simulink model "prob49_e_integral"  (R2016b)
settings: Solver=ode4  StartTime=0.0  StopTime=500.0  FixedStep=0.001  RelTol=1e-3
values from neighbouring files (symbols this model uses):
  alfa = 1    [p49Consts.m]
  beta = 0.1    [p49Consts.m]    (also in task49.m)
  beta_g = 0.1    [p49Consts.m]
  Gamma = [10 0 0 ... (first row only)    [p49Consts.m]
  k = 5    [p49Consts.m]    (also in task49.m)
  lambda_0 = 4    [p49Consts.m]    (also in task49.m = 1)
  lambda_1 = 4    [p49Consts.m]    (also in task49.m = 1)
settings Model: Creator=Kristian  LastModifiedBy=Kristian

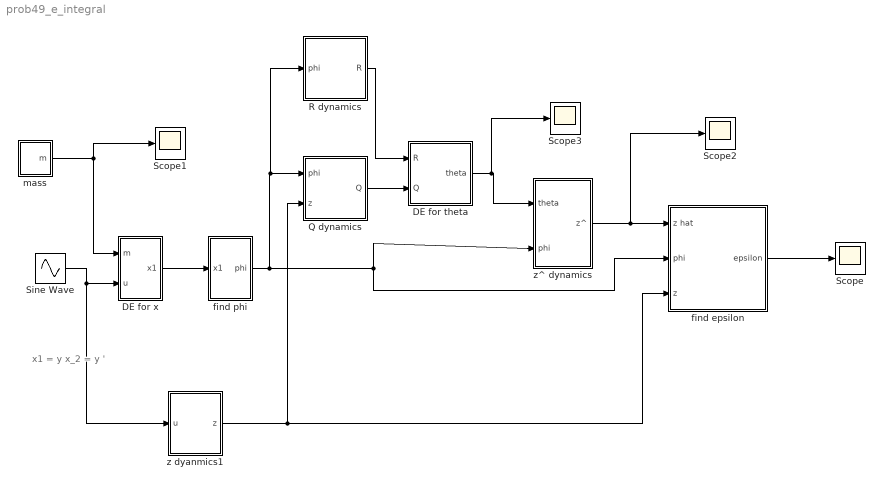
== system prob49_e_integral ==
  note: x1 = y
      | x_2 = y '
  DE for theta : Subsystem
  DE for x : Subsystem
  "Q dynamics " : Subsystem
  "R dynamics " : Subsystem
  Scope{,1..3} (4 alike) : Scope
  Sine Wave : Sin  Amplitude=5  Phase=0.3  SampleTime=0
  find epsilon : Subsystem
  find phi : Subsystem
  "mass " : Subsystem
  z dyanmics1 : Subsystem
  z^ dynamics : Subsystem
  wires:
  DE for x/1("x1 ") -> find phi/1(x1)
  find phi/1("phi ") -> "R dynamics "/1(phi), "Q dynamics "/1(phi), find epsilon/2(phi), z^ dynamics/2(phi)
  Sine Wave/1 -> z dyanmics1/1(u), DE for x/2(u)
  z^ dynamics/1("z^ ") -> Scope2/1, find epsilon/1(z hat)
  DE for theta/1("theta ") -> Scope3/1, z^ dynamics/1(theta)
  find epsilon/1("epsilon ") -> Scope/1
  z dyanmics1/1("z ") -> find epsilon/3(z), "Q dynamics "/2("z ")
  "Q dynamics "/1(Q) -> DE for theta/2(Q)
  "R dynamics "/1("R ") -> DE for theta/1("R ")
  "mass "/1(m) -> Scope1/1, DE for x/1("m ")

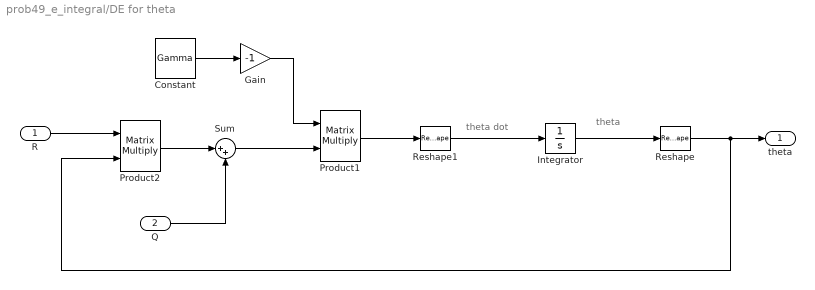
== system prob49_e_integral/DE for theta ==
  note: theta
  note: theta dot
  "R " : Inport
  Q : Inport  Port=2
  Constant : Constant  Value=Gamma  VectorParams1D=off
  Gain : Gain  Gain=-1
  Integrator : Integrator
  Product1 : Product  Multiplication=Matrix(*)
  Product2 : Product  Multiplication=Matrix(*)
  Reshape : Reshape  OutputDimensionality=Column vector (2-D)
  Reshape1 : Reshape  OutputDimensionality=Column vector (2-D)
  Sum : Sum  Inputs=|++
  "theta " : Outport
  wires:
  Integrator/1 -> Reshape/1
  Constant/1 -> Gain/1
  Product1/1 -> Reshape1/1
  Reshape1/1 -> Integrator/1
  Gain/1 -> Product1/1
  "R "/1 -> Product2/1
  Reshape/1 -> Product2/2, "theta "/1
  Product2/1 -> Sum/1
  Q/1 -> Sum/2
  Sum/1 -> Product1/2

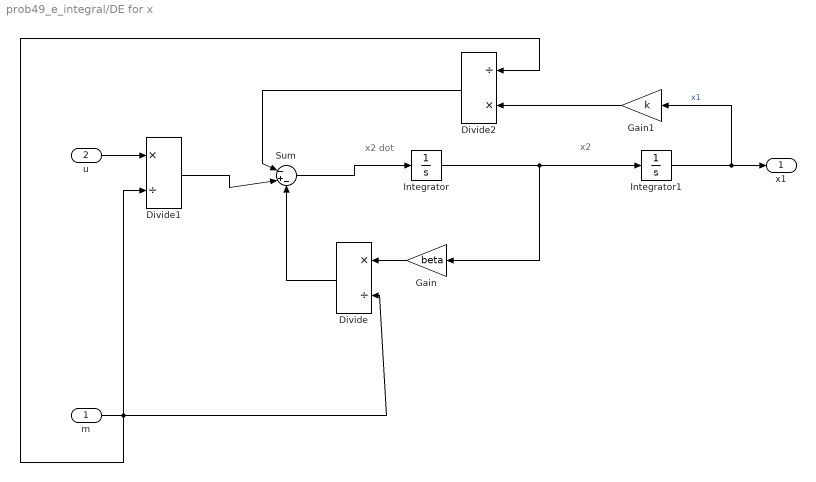
== system prob49_e_integral/DE for x ==
  note: x2 dot
  note: x2
  "m " : Inport
  u : Inport  Port=2
  Divide : Product  Inputs=*/
  Divide1 : Product  Inputs=*/
  Divide2 : Product  Inputs=/*
  Gain : Gain  Gain=beta
  Gain1 : Gain  Gain=k
  Integrator : Integrator
  Integrator1 : Integrator
  Sum : Sum  Inputs=|-+-
  "x1 " : Outport
  wires:
  Integrator/1 -> Integrator1/1, Gain/1
  Sum/1 -> Integrator/1
  Integrator1/1 -> Gain1/1, "x1 "/1  "x1"
  Gain/1 -> Divide/1
  "m "/1 -> Divide2/1, Divide/2, Divide1/2
  u/1 -> Divide1/1
  Gain1/1 -> Divide2/2
  Divide2/1 -> Sum/1
  Divide1/1 -> Sum/2
  Divide/1 -> Sum/3

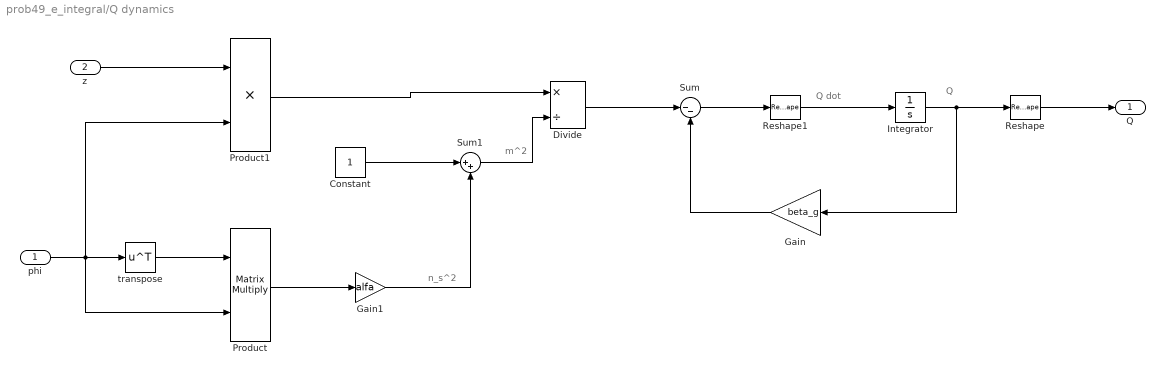
== system prob49_e_integral/Q dynamics  ==
  note: Q
  note: Q dot
  note: n_s^2
  note: m^2
  phi : Inport
  "z " : Inport  Port=2
  Constant : Constant
  Divide : Product  Inputs=*/
  Gain : Gain  Gain=beta_g
  Gain1 : Gain  Gain=alfa
  Integrator : Integrator
  Product : Product  Multiplication=Matrix(*)
  Product1 : Product
  Reshape : Reshape  OutputDimensionality=Column vector (2-D)
  Reshape1 : Reshape  OutputDimensionality=Column vector (2-D)
  Sum : Sum  Inputs=|--
  Sum1 : Sum  Inputs=|++
  transpose : Math  Operator=transpose  SaturateOnIntegerOverflow=on
  Q : Outport
  wires:
  Integrator/1 -> Gain/1, Reshape/1
  Reshape1/1 -> Integrator/1
  Reshape/1 -> Q/1
  Gain/1 -> Sum/2
  Sum/1 -> Reshape1/1
  Constant/1 -> Sum1/1
  transpose/1 -> Product/1
  Product/1 -> Gain1/1
  Gain1/1 -> Sum1/2
  phi/1 -> Product1/2, Product/2, transpose/1
  Product1/1 -> Divide/1
  Sum1/1 -> Divide/2
  Divide/1 -> Sum/1
  "z "/1 -> Product1/1

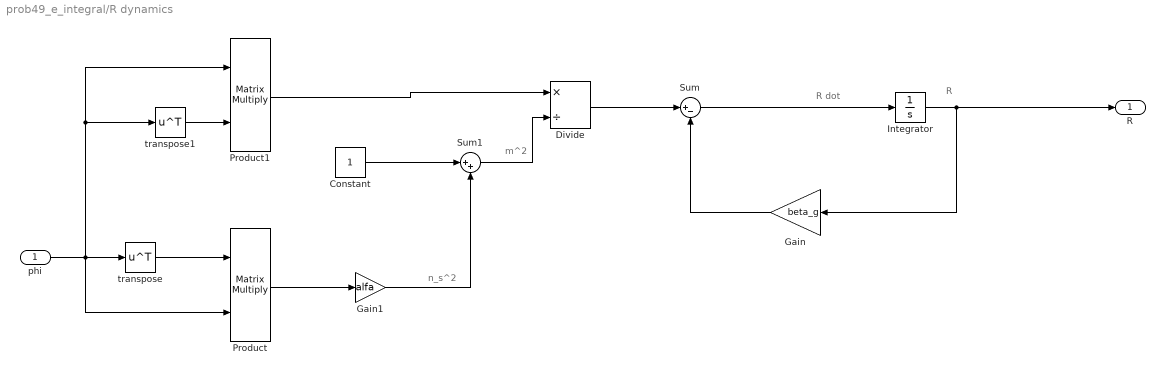
== system prob49_e_integral/R dynamics  ==
  note: R
  note: R dot
  note: n_s^2
  note: m^2
  phi : Inport
  Constant : Constant
  Divide : Product  Inputs=*/
  Gain : Gain  Gain=beta_g
  Gain1 : Gain  Gain=alfa
  Integrator : Integrator
  Product : Product  Multiplication=Matrix(*)
  Product1 : Product  Multiplication=Matrix(*)
  Sum : Sum  Inputs=|+-
  Sum1 : Sum  Inputs=|++
  transpose : Math  Operator=transpose  SaturateOnIntegerOverflow=on
  transpose1 : Math  Operator=transpose  SaturateOnIntegerOverflow=on
  "R " : Outport
  wires:
  Sum/1 -> Integrator/1
  Integrator/1 -> "R "/1, Gain/1
  Gain/1 -> Sum/2
  Constant/1 -> Sum1/1
  transpose/1 -> Product/1
  Product/1 -> Gain1/1
  Gain1/1 -> Sum1/2
  phi/1 -> transpose1/1, Product1/1, Product/2, transpose/1
  transpose1/1 -> Product1/2
  Product1/1 -> Divide/1
  Sum1/1 -> Divide/2
  Divide/1 -> Sum/1

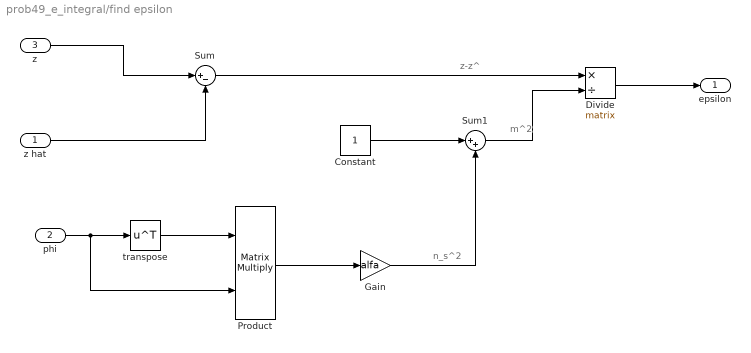
== system prob49_e_integral/find epsilon ==
  note: z-z^
  note: n_s^2
  note: m^2
  z hat : Inport
  phi : Inport  Port=2
  z : Inport  Port=3
  Constant : Constant
  Divide : Product  Inputs=*/  Multiplication=Matrix(*)
  Gain : Gain  Gain=alfa
  Product : Product  Multiplication=Matrix(*)
  Sum : Sum  Inputs=|+-
  Sum1 : Sum  Inputs=|++
  transpose : Math  Operator=transpose  SaturateOnIntegerOverflow=on
  "epsilon " : Outport
  wires:
  z/1 -> Sum/1
  z hat/1 -> Sum/2
  Constant/1 -> Sum1/1
  phi/1 -> Product/2, transpose/1
  transpose/1 -> Product/1
  Product/1 -> Gain/1
  Gain/1 -> Sum1/2
  Sum1/1 -> Divide/2
  Sum/1 -> Divide/1
  Divide/1 -> "epsilon "/1

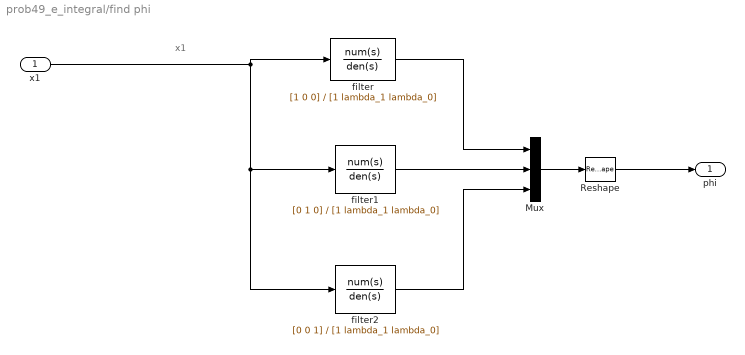
== system prob49_e_integral/find phi ==
  note: x1
  x1 : Inport
  Mux : Mux  Inputs=3
  Reshape : Reshape  OutputDimensionality=Column vector (2-D)
  filter : TransferFcn  Numerator=[1 0 0]  Denominator=[1 lambda_1 lambda_0]
  filter1 : TransferFcn  Numerator=[0 1 0]  Denominator=[1 lambda_1 lambda_0]
  filter2 : TransferFcn  Numerator=[0 0 1]  Denominator=[1 lambda_1 lambda_0]
  "phi " : Outport
  wires:
  x1/1 -> filter/1, filter2/1, filter1/1
  filter/1 -> Mux/1
  filter1/1 -> Mux/2
  filter2/1 -> Mux/3
  Mux/1 -> Reshape/1
  Reshape/1 -> "phi "/1

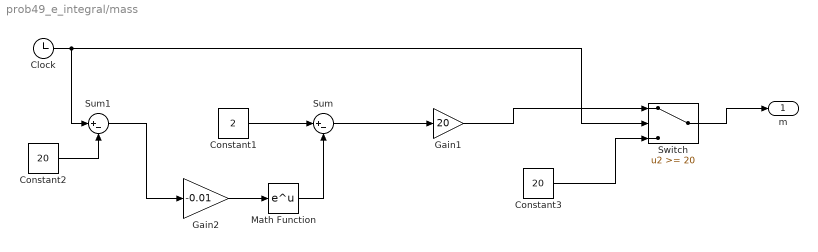
== system prob49_e_integral/mass  ==
  Clock : Clock
  Constant1 : Constant  Value=2
  Constant2 : Constant  Value=20
  Constant3 : Constant  Value=20
  Gain1 : Gain  Gain=20
  Gain2 : Gain  Gain=-0.01
  Math Function : Math  SaturateOnIntegerOverflow=on
  Sum : Sum  Inputs=|+-
  Sum1 : Sum  Inputs=|+-
  Switch : Switch  Threshold=20
  m : Outport
  wires:
  Clock/1 -> Sum1/1, Switch/2
  Switch/1 -> m/1
  Constant3/1 -> Switch/3
  Sum/1 -> Gain1/1
  Math Function/1 -> Sum/2
  Constant1/1 -> Sum/1
  Gain1/1 -> Switch/1
  Gain2/1 -> Math Function/1
  Constant2/1 -> Sum1/2
  Sum1/1 -> Gain2/1

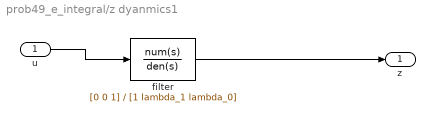
== system prob49_e_integral/z dyanmics1 ==
  u : Inport
  filter : TransferFcn  Numerator=[0 0 1]  Denominator=[1 lambda_1 lambda_0]
  "z " : Outport
  wires:
  u/1 -> filter/1
  filter/1 -> "z "/1

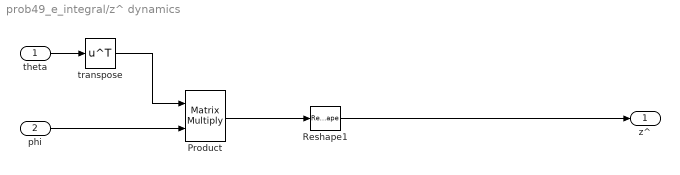
== system prob49_e_integral/z^ dynamics ==
  theta : Inport
  phi : Inport  Port=2
  Product : Product  Multiplication=Matrix(*)
  Reshape1 : Reshape  OutputDimensionality=Column vector (2-D)
  transpose : Math  Operator=transpose  SaturateOnIntegerOverflow=on
  "z^ " : Outport
  wires:
  Reshape1/1 -> "z^ "/1
  Product/1 -> Reshape1/1
  theta/1 -> transpose/1
  transpose/1 -> Product/1
  phi/1 -> Product/2
